simulink library "aerolibasang"  (Simulink 5.0)
values from neighbouring files (symbols this model uses):
  s = aeroliblist    [asbhelp.m]
undefined symbols (not defined in the file or in its folder): aeroassertmsg, data, kg, m, vel_case
libraries: simulink x8, aerolibconvert x7, aerolibasang x6
settings Model: Creator=sgage  LastModifiedBy=sgage  ExtModeAutoUpdateStatusClock=off

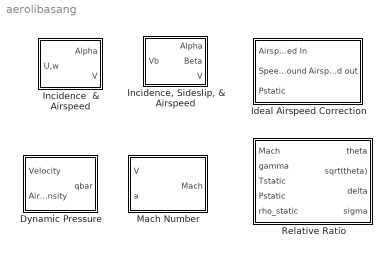
== system aerolibasang ==
  Dynamic Pressure : Subsystem
      mask Type: Dynamic Pressure
      mask Description: Compute dynamic pressure using velocity and air density.
      mask Help: web(asbhelp);
      mask Display:
      | port_label('input',1,'V','texmode','on');
      | port_label('input',2,'\rho','texmode','on');
      | port_label('output',1,'q','texmode','on');
      | disp('^1/_2 \rhoV^2','texmode','on');
  Ideal Airspeed Correction : Subsystem  mask(Ideal Airspeed Correction){units=Metric (MKS), vel_in=TAS, vel_out_tas=CAS, vel_out_eas=CAS, vel_out_cas=TAS, action=Error}
      mask prompts: vel_in "Airspeed input:"; vel_out_tas "Airspeed output:"; vel_out_eas "Airspeed output:"; vel_out_cas "Airspeed output:"; action "Action for out of range input:"
      mask help:
      | Calculate equivalent airspeed (EAS), calibrated airspeed (CAS), or true airspeed (TAS) from one of the other two airspeeds.
      |
      | Based on assumption of compressible, isentropic (subsonic flow), dry air with constant specific heat ratio (gamma).
      mask init:
      | [vel_case,ports,data] = aeroicon('aeroblkascorr','icon');
      | a0=340.2941;
      mask Help: web(asbhelp('idealairspeedcorrection'));
      mask StyleString: popup(Metric (MKS)|English (Velocity in ft/s)|English (Velocity in kts)),popup(TAS|EAS|CAS),popup(EAS|CAS),popup(TAS|CAS),popup(TAS|EAS),popup(None|Warning|Error)
      mask CallbackString: aeroicon('aeroblkascorr');|aeroicon('aeroblkascorr');||||
      mask Display:
      | port_label(ports(1).type,ports(1).port,ports(1).txt,'texmode','on');
      | port_label(ports(2).type,ports(2).port,ports(2).txt,'texmode','on');
      | port_label(ports(3).type,ports(3).port,ports(3).txt,'texmode','on');
      | port_label(ports(4).type,ports(4).port,ports(4).txt,'texmode','on');
  Incidence  & Airspeed : Subsystem
      mask Type: Incidence&Airspeed
      mask Description: Calculate the angle between the body and the velocity vector (incidence) and the velocity magnitude from the components in body axes (U,w).
      mask Help: web(asbhelp('incidenceairspeed'));
      mask Display:
      | port_label('input',1,'U, w','texmode','on');
      | port_label('output',1,'{\alpha}','texmode','on');
      | port_label('output',2,'V','texmode','on');
  "Incidence, Sideslip, & Airspeed" : Subsystem
      mask Type: Incidence,Sideslip,&Airspeed
      mask Description: Calculate the angles between the body and the velocity vector (incidence and sideslip), and the velocity magnitude from the components in body axes (Vb).
      mask Help: web(asbhelp('incidence'));
      mask Display:
      | port_label('input',1,'V_b','texmode','on');
      | port_label('output',1,'\alpha','texmode','on');
      | port_label('output',2,'\beta','texmode','on');
      | port_label('output',3,'V','texmode','on');
  Mach Number : Subsystem
      mask Type: Mach Number
      mask Description: Compute Mach number using velocity and speed of sound.
      mask Help: web(asbhelp);
      mask Display:
      | port_label('input',1,'V','texmode','on');
      | port_label('input',2,'a','texmode','on');
      | port_label('output',1,'Mach','texmode','on');
  Relative Ratio : Subsystem  mask(Relative Ratio){units=Metric (MKS), theta=on, sq_theta=on, delta=on, sigma=on}
      mask prompts: sq_theta "Square root of theta:"
      mask help:
      | Calculate the relative atmospheric ratios including relative temperature ratio (theta), square root of theta, relative pressure ratio (delta), and relative density ratio (sigma).
      |
      | Theta represents the ratio of the air stream temperature at a chosen reference station relative to sea level standard atmospheric conditions.
      |
      | Delta represents the ratio of the air stream pressure at a chosen reference station relative to sea level standard atmospheric conditions.
      |
      | Sigma represents the ratio of the air stream density at a chosen reference station relative to sea level standard atmospheric conditions.
      mask init:
      | ports = aeroicon('aeroblkratio','icon');
      mask Help: web(asbhelp('relativeratio'));
      mask StyleString: popup(Metric (MKS)|English),checkbox,checkbox,checkbox,checkbox
      mask CallbackString:
      | |aeroicon('aeroblkratio','','theta');
      | |aeroicon('aeroblkratio','','sq_theta');
      | 
      | |aeroicon('aeroblkratio','','delta');
      | 
      | |aeroicon('aeroblkratio','','sigma');
      mask Display:
      | port_label(ports(1).type,ports(1).port,ports(1).txt,'texmode','on');
      | port_label(ports(2).type,ports(2).port,ports(2).txt,'texmode','on');
      | port_label(ports(3).type,ports(3).port,ports(3).txt,'texmode','on');
      | port_label(ports(4).type,ports(4).port,ports(4).txt,'texmode','on');
      | port_label(ports(5).type,ports(5).port,ports(5).txt,'texmode','on');
      | port_label(ports(6).type,ports(6).port,ports(6).txt,'texmode','on');
      | port_label(ports(7).type,ports(7).port,ports(7).txt,'texmode','on');
      | port_label(ports(8).type,ports(8).port,ports(8).txt,'texmode','on');
      | port_label(ports(9).type,ports(9).port,ports(9).txt,'texmode','on');

== system aerolibasang/Dynamic Pressure ==
  Velocity : Inport
  Air Density : Inport  Port=2
  1/2rhoV^2 : Gain  Gain=1/2  SaturateOnIntegerOverflow=on
  Dot Product : simulink/Math Operations/Dot Product
  Product2 : Product  SaturateOnIntegerOverflow=on  InputSameDT=on
  qbar : Outport  InitialOutput=0
  wires:
  Velocity/1 -> Dot Product/2, Dot Product/1
  Dot Product/1 -> Product2/1
  Air Density/1 -> Product2/2
  Product2/1 -> 1/2rhoV^2/1
  1/2rhoV^2/1 -> qbar/1

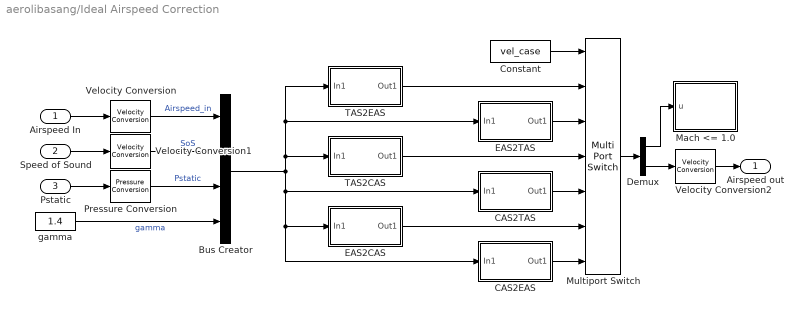
== system aerolibasang/Ideal Airspeed Correction ==
  Airspeed In : Inport
  Speed of Sound : Inport  Port=2
  Pstatic : Inport  Port=3
  Bus Creator : BusCreator
  CAS2EAS : Subsystem  TreatAsAtomicUnit=on
  CAS2TAS : Subsystem  TreatAsAtomicUnit=on
  Constant : Constant  Value=vel_case  ShowAdditionalParam=on
  Demux : Demux  Outputs=2
  EAS2CAS : Subsystem  TreatAsAtomicUnit=on
  EAS2TAS : Subsystem  TreatAsAtomicUnit=on
  Mach <= 1.0 : Subsystem  Description=u <= 1.0  mask(Checks_SMax){max=1.0, max_included=on, enabled=on, callback=aeroassertmsg('aeroblkascorr'), stopWhenAssertionFail=on, export=off, icon=graphic}
      mask prompts: max "Upper bound:"; max_included "Inclusive boundary"; enabled "Enable assertion"; callback "Simulation callback when assertion fails (optional):"; stopWhenAssertionFail "Stop simulation when assertion fails"; export "Output assertion signal"; icon "Select icon type:"
      mask help: Assert that the input signal is less than (or optionally equal to) a static upper bound.
      mask init:
      | update_assert_sys(gcbh);
      mask StyleString: edit,checkbox,checkbox,edit,checkbox,checkbox,popup(graphic|text)
      mask Display: image(imread('Checks_SMax.bmp','bmp'),'center')
  Multiport Switch : MultiPortSwitch  Inputs=6  SaturateOnIntegerOverflow=on
  Pressure Conversion : aerolibconvert/Pressure Conversion  IU=Pa  OU=Pa
  TAS2CAS : Subsystem  TreatAsAtomicUnit=on
  TAS2EAS : Subsystem  TreatAsAtomicUnit=on
  Velocity Conversion : aerolibconvert/Velocity Conversion  IU=m/s  OU=m/s
  Velocity Conversion1 : aerolibconvert/Velocity Conversion  IU=m/s  OU=m/s
  Velocity Conversion2 : aerolibconvert/Velocity Conversion  IU=m/s  OU=m/s
  gamma : Constant  Value=1.4  ShowAdditionalParam=on
  Airspeed out : Outport
  wires:
  gamma/1 -> Bus Creator/4  "gamma"
  EAS2CAS/1(Out1) -> Multiport Switch/6
  TAS2CAS/1(Out1) -> Multiport Switch/4
  CAS2EAS/1(Out1) -> Multiport Switch/7
  CAS2TAS/1(Out1) -> Multiport Switch/5
  TAS2EAS/1(Out1) -> Multiport Switch/2
  Bus Creator/1 -> TAS2CAS/1(In1), EAS2CAS/1(In1), CAS2EAS/1(In1), CAS2TAS/1(In1), TAS2EAS/1(In1), EAS2TAS/1(In1)
  Multiport Switch/1 -> Demux/1
  Velocity Conversion2/1 -> Airspeed out/1
  Velocity Conversion1/1 -> Bus Creator/2  "SoS"
  Velocity Conversion/1 -> Bus Creator/1  "Airspeed_in"
  Pressure Conversion/1 -> Bus Creator/3  "Pstatic"
  Pstatic/1 -> Pressure Conversion/1
  Speed of Sound/1 -> Velocity Conversion1/1
  Airspeed In/1 -> Velocity Conversion/1
  Constant/1 -> Multiport Switch/1
  EAS2TAS/1(Out1) -> Multiport Switch/3
  Demux/2 -> Velocity Conversion2/1
  Demux/1 -> Mach <= 1.0/1(u)

== system aerolibasang/Incidence  & Airspeed ==
  U,w : Inport
  Airspeed : Math  Operator=sqrt
  Demux : Demux  Outputs=2
  Dot Product : simulink/Math Operations/Dot Product  OutDataType=sfix(16)  OutScaling=2^-10  DoSatur=off
  Incidence : Trigonometry  Operator=atan2
  Alpha : Outport  InitialOutput=0
  V : Outport  Port=2  InitialOutput=0
  wires:
  Airspeed/1 -> V/1
  Incidence/1 -> Alpha/1
  U,w/1 -> Dot Product/1, Dot Product/2, Demux/1
  Dot Product/1 -> Airspeed/1
  Demux/1 -> Incidence/2
  Demux/2 -> Incidence/1

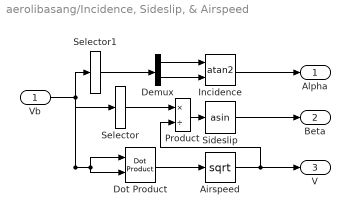
== system aerolibasang/Incidence, Sideslip, & Airspeed ==
  Vb : Inport
  Airspeed : Math  Operator=sqrt
  Demux : Demux  Outputs=2
  Dot Product : simulink/Math Operations/Dot Product
  Incidence : Trigonometry  Operator=atan2
  Product : Product  Inputs=*/  SaturateOnIntegerOverflow=on
  Selector : Selector  Elements=2  InputPortWidth=3
  Selector1 : Selector  Elements=[3 1]  InputPortWidth=3
  Sideslip : Trigonometry  Operator=asin
  Alpha : Outport  InitialOutput=0
  Beta : Outport  Port=2  InitialOutput=0
  V : Outport  Port=3  InitialOutput=0
  wires:
  Selector/1 -> Product/1
  Sideslip/1 -> Beta/1
  Vb/1 -> Selector/1, Dot Product/2, Dot Product/1, Selector1/1
  Incidence/1 -> Alpha/1
  Airspeed/1 -> V/1, Product/2
  Dot Product/1 -> Airspeed/1
  Selector1/1 -> Demux/1
  Demux/2 -> Incidence/2
  Demux/1 -> Incidence/1
  Product/1 -> Sideslip/1

== system aerolibasang/Mach Number ==
  V : Inport
  a : Inport  Port=2
  Dot Product : simulink/Math Operations/Dot Product
  Product1 : Product  Inputs=*/  SaturateOnIntegerOverflow=on  InputSameDT=on
  vt : Math  Operator=sqrt
  Mach : Outport
  wires:
  V/1 -> Dot Product/2, Dot Product/1
  a/1 -> Product1/2
  vt/1 -> Product1/1
  Product1/1 -> Mach/1
  Dot Product/1 -> vt/1

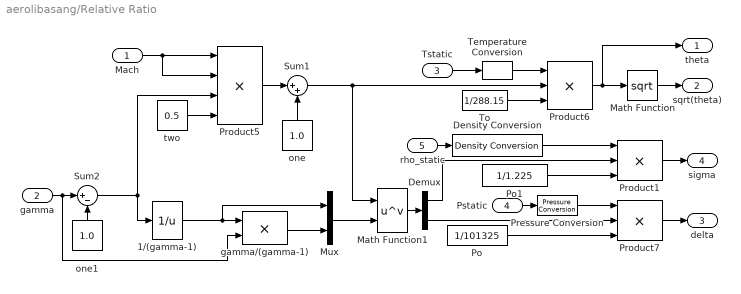
== system aerolibasang/Relative Ratio ==
  Mach : Inport
  gamma : Inport  Port=2
  Tstatic : Inport  Port=3
  Pstatic : Inport  Port=4
  rho_static : Inport  Port=5
  1/(gamma-1) : Math  Operator=reciprocal
  Demux : Demux  Outputs=2
  Density Conversion : aerolibconvert/Density Conversion  IU=kg/m^3  OU=kg/m^3
  Math Function : Math  Operator=sqrt
  Math Function1 : Math  Operator=pow
  Mux : Mux  Inputs=2
  Po : Constant  Value=1/101325  ShowAdditionalParam=on
  Po1 : Constant  Value=1/1.225  ShowAdditionalParam=on
  Pressure Conversion : aerolibconvert/Pressure Conversion  IU=Pa  OU=Pa
  Product1 : Product  Inputs=3  ShowAdditionalParam=on  SaturateOnIntegerOverflow=on  InputSameDT=on
  Product5 : Product  Inputs=4  SaturateOnIntegerOverflow=on  InputSameDT=on
  Product6 : Product  Inputs=3  ShowAdditionalParam=on  SaturateOnIntegerOverflow=on  InputSameDT=on
  Product7 : Product  Inputs=3  ShowAdditionalParam=on  SaturateOnIntegerOverflow=on  InputSameDT=on
  Sum1 : Sum  Inputs=|++  SaturateOnIntegerOverflow=on  InputSameDT=on
  Sum2 : Sum  Inputs=|+-  ShowAdditionalParam=on  SaturateOnIntegerOverflow=on  InputSameDT=on
  Temperature Conversion : aerolibconvert/Temperature Conversion  IU=K  OU=K
  To : Constant  Value=1/288.15  ShowAdditionalParam=on
  gamma/(gamma-1) : Product  SaturateOnIntegerOverflow=on
  one : Constant  Orientation=up  Value=1.0  ShowAdditionalParam=on
  one1 : Constant  Orientation=up  Value=1.0  ShowAdditionalParam=on
  two : Constant  Value=0.5  ShowAdditionalParam=on
  theta : Outport
  sqrt(theta) : Outport  Port=2
  delta : Outport  Port=3
  sigma : Outport  Port=4
  wires:
  Mux/1 -> Math Function1/2
  gamma/(gamma-1)/1 -> Mux/2
  1/(gamma-1)/1 -> Mux/1, gamma/(gamma-1)/1
  Sum2/1 -> 1/(gamma-1)/1, Product5/3
  one1/1 -> Sum2/2
  gamma/1 -> gamma/(gamma-1)/2, Sum2/1
  Temperature Conversion/1 -> Product6/1
  Tstatic/1 -> Temperature Conversion/1
  Math Function/1 -> sqrt(theta)/1
  Product6/1 -> Math Function/1, theta/1
  To/1 -> Product6/3
  Demux/1 -> Product1/2
  Math Function1/1 -> Demux/1
  Pressure Conversion/1 -> Product7/1
  Pstatic/1 -> Pressure Conversion/1
  Po/1 -> Product7/3
  Demux/2 -> Product7/2
  Product7/1 -> delta/1
  two/1 -> Product5/4
  Product5/1 -> Sum1/1
  one/1 -> Sum1/2
  Sum1/1 -> Product6/2, Math Function1/1
  Mach/1 -> Product5/1, Product5/2
  Po1/1 -> Product1/3
  Product1/1 -> sigma/1
  rho_static/1 -> Density Conversion/1
  Density Conversion/1 -> Product1/1

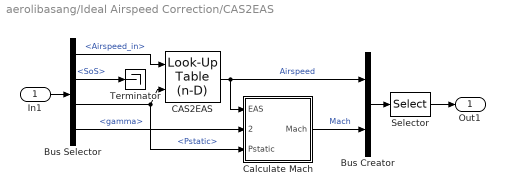
== system aerolibasang/Ideal Airspeed Correction/CAS2EAS ==
  In1 : Inport
  Bus Creator : BusCreator  Inputs=2
  Bus Selector : BusSelector  OutputSignals=Airspeed_in,SoS,Pstatic,gamma
  CAS2EAS : simulink/Look-Up Tables/Look-Up Table (n-D)  numDimsPopupSelect=2  bp1=data.aeroasV_bp  bp2=data.aeroasP_bp  bp3=[1:3]  bp4=[1:3]  bpcell={ [1:3], [1:3] }  explicitNumDims=2  searchMode=Linear Search  cacheBpFlag=on  vectorInputFlag=off  tableData=[data.aeroasVe_table]'  interpMethod=Cubic Spline  extrapMethod=Cubic Spline  rangeErrorMode=None
  Calculate Mach : Subsystem
  Selector : Selector  Elements=[2 1]  InputPortWidth=2
  Terminator : Terminator
  Out1 : Outport
  wires:
  CAS2EAS/1 -> Calculate Mach/1(EAS), Bus Creator/1  "Airspeed"
  Bus Selector/2 -> Terminator/1  "<SoS>"
  Bus Selector/1 -> CAS2EAS/1  "<Airspeed_in>"
  Bus Selector/3 -> CAS2EAS/2, Calculate Mach/3(Pstatic)  "<Pstatic>"
  In1/1 -> Bus Selector/1
  Bus Selector/4 -> Calculate Mach/2(gamma)  "<gamma>"
  Calculate Mach/1(Mach) -> Bus Creator/2  "Mach"
  Bus Creator/1 -> Selector/1
  Selector/1 -> Out1/1

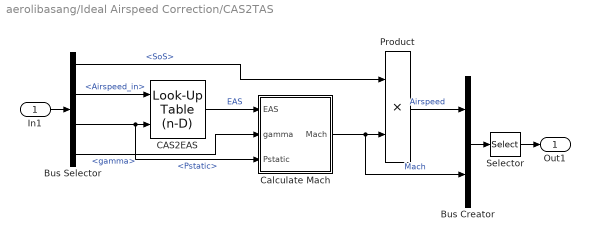
== system aerolibasang/Ideal Airspeed Correction/CAS2TAS ==
  In1 : Inport
  Bus Creator : BusCreator  Inputs=2
  Bus Selector : BusSelector  OutputSignals=SoS,Airspeed_in,Pstatic,gamma
  CAS2EAS : simulink/Look-Up Tables/Look-Up Table (n-D)  numDimsPopupSelect=2  bp1=data.aeroasV_bp  bp2=data.aeroasP_bp  bp3=[1:3]  bp4=[1:3]  bpcell={ [1:3], [1:3] }  explicitNumDims=2  searchMode=Linear Search  cacheBpFlag=on  vectorInputFlag=off  tableData=[data.aeroasVe_table]'  interpMethod=Cubic Spline  extrapMethod=Cubic Spline  rangeErrorMode=None
  Calculate Mach : Subsystem
  Product : Product  SaturateOnIntegerOverflow=on
  Selector : Selector  Elements=[2 1]  InputPortWidth=2
  Out1 : Outport
  wires:
  Calculate Mach/1(Mach) -> Product/2, Bus Creator/2  "Mach"
  Bus Selector/4 -> Calculate Mach/2(gamma)  "<gamma>"
  Product/1 -> Bus Creator/1  "Airspeed"
  Bus Selector/1 -> Product/1  "<SoS>"
  Bus Selector/2 -> CAS2EAS/1  "<Airspeed_in>"
  In1/1 -> Bus Selector/1
  Bus Selector/3 -> CAS2EAS/2, Calculate Mach/3(Pstatic)  "<Pstatic>"
  CAS2EAS/1 -> Calculate Mach/1(EAS)  "EAS"
  Bus Creator/1 -> Selector/1
  Selector/1 -> Out1/1

== system aerolibasang/Ideal Airspeed Correction/EAS2CAS ==
  In1 : Inport
  Bus Creator : BusCreator  Inputs=2
  Bus Selector : BusSelector  OutputSignals=Airspeed_in,gamma,Pstatic,SoS
  Calculate Mach : Subsystem
  EAS2CAS : simulink/Look-Up Tables/Look-Up Table (n-D)  numDimsPopupSelect=2  bp1=data.aeroasV_bp  bp2=data.aeroasP_bp  bp3=[1:3]  bp4=[1:3]  bpcell={ [1:3], [1:3] }  explicitNumDims=2  searchMode=Linear Search  cacheBpFlag=on  vectorInputFlag=off  tableData=[data.aeroasVc_table]'  interpMethod=Cubic Spline  extrapMethod=Cubic Spline  rangeErrorMode=None
  Terminator : Terminator
  Out1 : Outport
  wires:
  Bus Selector/1 -> EAS2CAS/1, Calculate Mach/1(EAS)  "<Airspeed_in>"
  Bus Selector/4 -> Terminator/1  "<SoS>"
  Bus Selector/3 -> EAS2CAS/2, Calculate Mach/3(Pstatic)  "<Pstatic>"
  In1/1 -> Bus Selector/1
  EAS2CAS/1 -> Bus Creator/2  "Airspeed"
  Bus Selector/2 -> Calculate Mach/2(gamma)  "<gamma>"
  Calculate Mach/1(Mach) -> Bus Creator/1  "Mach"
  Bus Creator/1 -> Out1/1

== system aerolibasang/Ideal Airspeed Correction/EAS2TAS ==
  In1 : Inport
  Bus Creator : BusCreator  Inputs=2
  Bus Selector : BusSelector  OutputSignals=SoS,Airspeed_in,gamma,Pstatic
  Calculate Mach : Subsystem
  Product : Product  SaturateOnIntegerOverflow=on
  Selector : Selector  Elements=[2 1]  InputPortWidth=2
  Out1 : Outport
  wires:
  Product/1 -> Bus Creator/1  "Airspeed"
  Bus Selector/4 -> Calculate Mach/3(Pstatic)  "<Pstatic>"
  Calculate Mach/1(Mach) -> Product/2, Bus Creator/2  "Mach"
  Bus Selector/1 -> Product/1  "<SoS>"
  In1/1 -> Bus Selector/1
  Bus Selector/3 -> Calculate Mach/2(gamma)  "<gamma>"
  Bus Selector/2 -> Calculate Mach/1(EAS)  "<Airspeed_in>"
  Bus Creator/1 -> Selector/1
  Selector/1 -> Out1/1

== system aerolibasang/Ideal Airspeed Correction/Mach <= 1.0 ==
  u : Inport
  Assertion : Assertion  AssertionFailFcn=aeroassertmsg('aeroblkascorr')
  max_relop : RelationalOperator  Operator=<=  InputSameDT=on
  max_val : Constant  Value=max
  mintype : DataTypeConversion  SaturateOnIntegerOverflow=on
  out : Terminator
  wires:
  mintype/1 -> max_relop/2
  u/1 -> max_relop/1
  max_val/1 -> mintype/1
  max_relop/1 -> Assertion/1, out/1

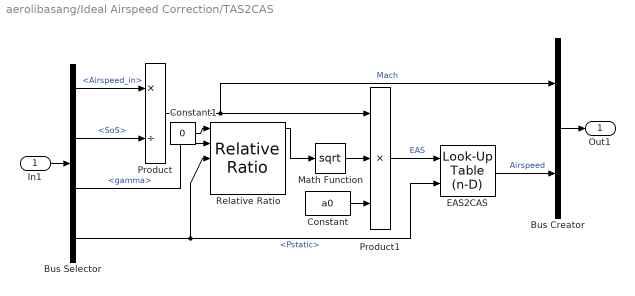
== system aerolibasang/Ideal Airspeed Correction/TAS2CAS ==
  In1 : Inport
  Bus Creator : BusCreator  Inputs=2
  Bus Selector : BusSelector  OutputSignals=Airspeed_in,SoS,gamma,Pstatic
  Constant : Constant  Value=a0  ShowAdditionalParam=on
  Constant1 : Constant  Value=0  ShowAdditionalParam=on
  EAS2CAS : simulink/Look-Up Tables/Look-Up Table (n-D)  numDimsPopupSelect=2  bp1=data.aeroasV_bp  bp2=data.aeroasP_bp  bp3=[1:3]  bp4=[1:3]  bpcell={ [1:3], [1:3] }  explicitNumDims=2  searchMode=Linear Search  cacheBpFlag=on  vectorInputFlag=off  tableData=[data.aeroasVc_table]'  interpMethod=Cubic Spline  extrapMethod=Cubic Spline  rangeErrorMode=None
  Math Function : Math  Operator=sqrt
  Product : Product  Inputs=*/  SaturateOnIntegerOverflow=on
  Product1 : Product  Inputs=3  SaturateOnIntegerOverflow=on
  Relative Ratio : aerolibasang/Relative Ratio  units=Metric (MKS)  theta=off  sq_theta=off  delta=on  sigma=off
  Out1 : Outport
  wires:
  Bus Selector/3 -> Relative Ratio/2  "<gamma>"
  Constant1/1 -> Relative Ratio/1
  Product1/1 -> EAS2CAS/1  "EAS"
  Constant/1 -> Product1/3
  Math Function/1 -> Product1/2
  Relative Ratio/1 -> Math Function/1
  Product/1 -> Product1/1, Bus Creator/1  "Mach"
  Bus Selector/2 -> Product/2  "<SoS>"
  Bus Selector/1 -> Product/1  "<Airspeed_in>"
  Bus Selector/4 -> EAS2CAS/2, Relative Ratio/3  "<Pstatic>"
  EAS2CAS/1 -> Bus Creator/2  "Airspeed"
  In1/1 -> Bus Selector/1
  Bus Creator/1 -> Out1/1

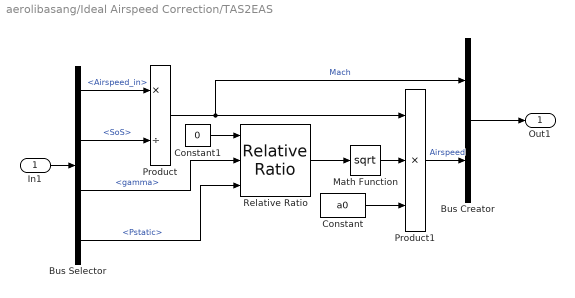
== system aerolibasang/Ideal Airspeed Correction/TAS2EAS ==
  In1 : Inport
  Bus Creator : BusCreator  Inputs=2
  Bus Selector : BusSelector  OutputSignals=Airspeed_in,SoS,gamma,Pstatic
  Constant : Constant  Value=a0  ShowAdditionalParam=on
  Constant1 : Constant  Value=0  ShowAdditionalParam=on
  Math Function : Math  Operator=sqrt
  Product : Product  Inputs=*/  SaturateOnIntegerOverflow=on
  Product1 : Product  Inputs=3  SaturateOnIntegerOverflow=on
  Relative Ratio : aerolibasang/Relative Ratio  units=Metric (MKS)  theta=off  sq_theta=off  delta=on  sigma=off
  Out1 : Outport
  wires:
  Bus Selector/3 -> Relative Ratio/2  "<gamma>"
  Constant1/1 -> Relative Ratio/1
  Product1/1 -> Bus Creator/2  "Airspeed"
  Constant/1 -> Product1/3
  Math Function/1 -> Product1/2
  Relative Ratio/1 -> Math Function/1
  Product/1 -> Product1/1, Bus Creator/1  "Mach"
  Bus Selector/2 -> Product/2  "<SoS>"
  Bus Selector/1 -> Product/1  "<Airspeed_in>"
  Bus Selector/4 -> Relative Ratio/3  "<Pstatic>"
  In1/1 -> Bus Selector/1
  Bus Creator/1 -> Out1/1

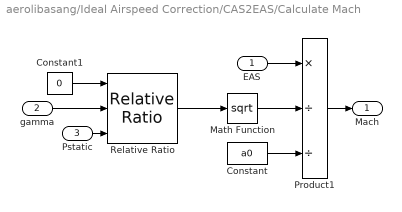
== system aerolibasang/Ideal Airspeed Correction/CAS2EAS/Calculate Mach ==
  EAS : Inport
  gamma : Inport  Port=2
  Pstatic : Inport  Port=3
  Constant : Constant  Value=a0  ShowAdditionalParam=on
  Constant1 : Constant  Value=0  ShowAdditionalParam=on
  Math Function : Math  Operator=sqrt
  Product1 : Product  Inputs=*//  SaturateOnIntegerOverflow=on
  Relative Ratio : aerolibasang/Relative Ratio  units=Metric (MKS)  theta=off  sq_theta=off  delta=on  sigma=off
  Mach : Outport
  wires:
  Constant1/1 -> Relative Ratio/1
  Constant/1 -> Product1/3
  Math Function/1 -> Product1/2
  Relative Ratio/1 -> Math Function/1
  EAS/1 -> Product1/1
  Pstatic/1 -> Relative Ratio/3
  Product1/1 -> Mach/1
  gamma/1 -> Relative Ratio/2

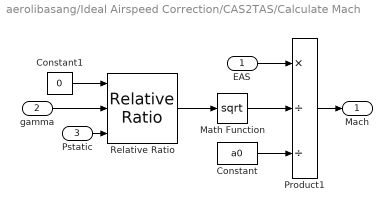
== system aerolibasang/Ideal Airspeed Correction/CAS2TAS/Calculate Mach ==
  EAS : Inport
  gamma : Inport  Port=2
  Pstatic : Inport  Port=3
  Constant : Constant  Value=a0  ShowAdditionalParam=on
  Constant1 : Constant  Value=0  ShowAdditionalParam=on
  Math Function : Math  Operator=sqrt
  Product1 : Product  Inputs=*//  SaturateOnIntegerOverflow=on
  Relative Ratio : aerolibasang/Relative Ratio  units=Metric (MKS)  theta=off  sq_theta=off  delta=on  sigma=off
  Mach : Outport
  wires:
  gamma/1 -> Relative Ratio/2
  Product1/1 -> Mach/1
  Pstatic/1 -> Relative Ratio/3
  EAS/1 -> Product1/1
  Relative Ratio/1 -> Math Function/1
  Math Function/1 -> Product1/2
  Constant/1 -> Product1/3
  Constant1/1 -> Relative Ratio/1

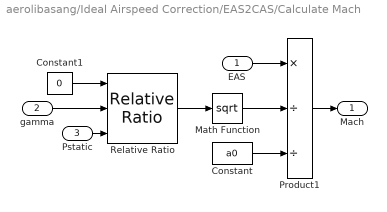
== system aerolibasang/Ideal Airspeed Correction/EAS2CAS/Calculate Mach ==
  EAS : Inport
  gamma : Inport  Port=2
  Pstatic : Inport  Port=3
  Constant : Constant  Value=a0  ShowAdditionalParam=on
  Constant1 : Constant  Value=0  ShowAdditionalParam=on
  Math Function : Math  Operator=sqrt
  Product1 : Product  Inputs=*//  SaturateOnIntegerOverflow=on
  Relative Ratio : aerolibasang/Relative Ratio  units=Metric (MKS)  theta=off  sq_theta=off  delta=on  sigma=off
  Mach : Outport
  wires:
  Constant1/1 -> Relative Ratio/1
  Constant/1 -> Product1/3
  Math Function/1 -> Product1/2
  Relative Ratio/1 -> Math Function/1
  EAS/1 -> Product1/1
  Pstatic/1 -> Relative Ratio/3
  Product1/1 -> Mach/1
  gamma/1 -> Relative Ratio/2

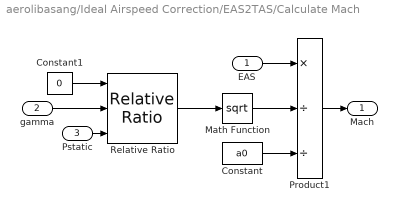
== system aerolibasang/Ideal Airspeed Correction/EAS2TAS/Calculate Mach ==
  EAS : Inport
  gamma : Inport  Port=2
  Pstatic : Inport  Port=3
  Constant : Constant  Value=a0  ShowAdditionalParam=on
  Constant1 : Constant  Value=0  ShowAdditionalParam=on
  Math Function : Math  Operator=sqrt
  Product1 : Product  Inputs=*//  SaturateOnIntegerOverflow=on
  Relative Ratio : aerolibasang/Relative Ratio  units=Metric (MKS)  theta=off  sq_theta=off  delta=on  sigma=off
  Mach : Outport
  wires:
  gamma/1 -> Relative Ratio/2
  Product1/1 -> Mach/1
  Pstatic/1 -> Relative Ratio/3
  EAS/1 -> Product1/1
  Relative Ratio/1 -> Math Function/1
  Math Function/1 -> Product1/2
  Constant/1 -> Product1/3
  Constant1/1 -> Relative Ratio/1
